simulink model "flightControlSystem"  (R2021a)
settings: Solver=ode3  StartTime=0  StopTime=TFinal  FixedStep=Ts  RelTol=1e-3  EnableMultiTasking=on
undefined symbols (not defined in the file): BINARIZER_THRESHOLD, codertarget, COG_X, COG_Y, Controller, DiscIntNeverNeededParam, Discrete, Estimator, FOV, g, G_B_GAIN, gray, init, MAX_RADIUS_CROWN, MIN_RADIUS_CROWN, S, Sensors, SQUARE_KERNEL, strel, Time, Ts, var_acc_angle_N, var_bias_gyr_N, var_gyro_p_N, Vehicle
libraries: simulink x38, slpidlib x4, ctrlSharedLib x4, sharedtransform x3, visionmorphops x2, radarlib x1, parrotlib x1
(part 3 of 3)

== matlab function flightControlSystem/Image Processing System/4dots picker/Trans_cordinate3 ==
  data: v input; y output; S parameter
function y = Trans_cordinate(v , S)
w = zeros(2,1);
w(1) = (S/2)-v(1);
w(2) = v(2)-S/2;
y = w;
